simulink model "Simulink_version_with_trivial_traj_reference"  (Simulink 7.5)
settings: Solver=ode5  StartTime=0.0  StopTime=10.0  FixedStep=0.02  RelTol=1e-3
values from neighbouring files (symbols this model uses):
  Kff = Kglob*Taeq + Gaeq    [Sim_LinRob_GlobMIMO_AxleTree.m]
undefined symbols (not defined in the file or in its folder): Kglob
libraries: simulink x2
settings Model: Creator=fclaveau  LastModifiedBy=fclaveau

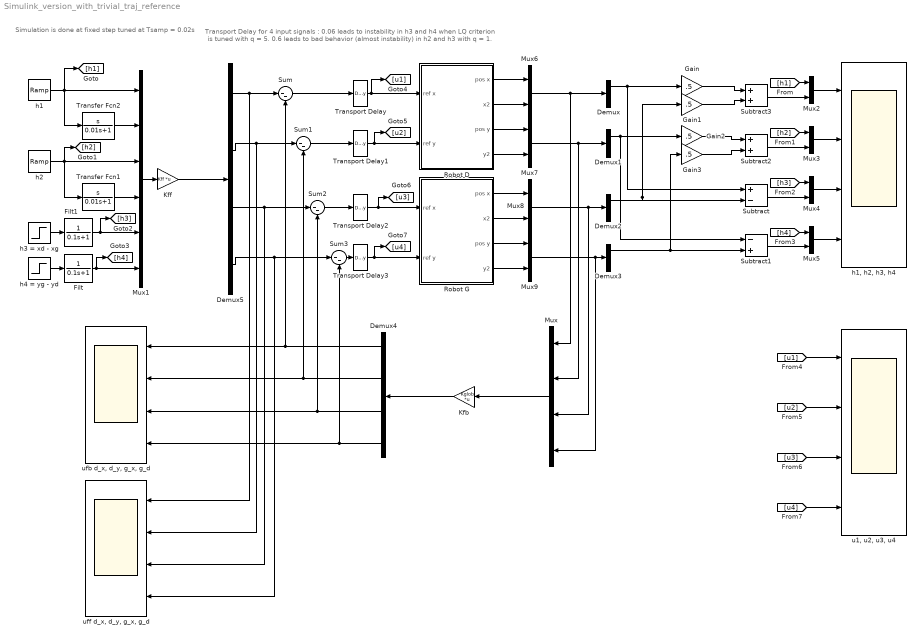
== system Simulink_version_with_trivial_traj_reference ==
  note: Transport Delay for 4 input signals :
      | 0.06 leads to instability in h3 and h4 when LQ criterion is tuned with q = 5.
      | 0.6 leads to bad behavior (almost instability) in h2 and h3 with q = 1.
  note: Simulation is done at fixed step
      | tuned at Tsamp = 0.02s
  Demux{,1..3} (4 alike) : Demux  Outputs=2
  Demux4 : Demux
  Demux5 : Demux
  Filt : TransferFcn  Denominator=[0.1 1]
  Filt1 : TransferFcn  Denominator=[0.1 1]
  Gain{,1..3} (4 alike) : Gain  Gain=.5  ParameterDataType=fixdt(1, 16)  ParameterScaling=2^0  OutDataType=fixdt(1, 16)  OutScaling=2^0
  Kfb : Gain  Gain=Kglob  Multiplication=Matrix(K*u)  ParameterDataType=fixdt(1, 16)  ParameterScaling=2^0  OutDataType=fixdt(1, 16)  OutScaling=2^0
  Kff : Gain  Gain=Kff  Multiplication=Matrix(K*u)  ParameterDataType=fixdt(1, 16)  ParameterScaling=2^0  OutDataType=fixdt(1, 16)  OutScaling=2^0
  Mux : Mux
  Mux1 : Mux  Inputs=6
  Mux{2..9} (8 alike) : Mux  Inputs=2
  Robot D : Subsystem
  Robot G : Subsystem
  Subtract : Sum  Inputs=+-  OutDataType=fixdt(1, 16)  OutScaling=2^-10
  Subtract1 : Sum  Inputs=-+  OutDataType=fixdt(1, 16)  OutScaling=2^-10
  Subtract2 : Sum  OutDataType=fixdt(1, 16)  OutScaling=2^-10
  Subtract3 : Sum  OutDataType=fixdt(1, 16)  OutScaling=2^-10
  Sum{,1..3} (4 alike) : Sum  Inputs=|--  OutDataType=fixdt(1, 16)  OutScaling=2^0
  Transfer Fcn1 : TransferFcn  Numerator=[1 0]  Denominator=[0.01 1]
  Transfer Fcn2 : TransferFcn  Numerator=[1 0]  Denominator=[0.01 1]
  Transport Delay{,1..3} (4 alike) : TransportDelay  DelayTime=0.6
  h1 : simulink/Sources/Ramp  SystemSampleTime=-1  slope=1  start=1  X0=0
  "h1, h2, h3, h4" : Scope  NumInputPorts=4
      settings: YMin=-5~-5~-5~-5  YMax=5~5~5~5
  h2 : simulink/Sources/Ramp  SystemSampleTime=-1  slope=1  start=3  X0=0
  h3 = xd - xg : Step  Time=5  After=2  SampleTime=0
  h4 = yg - yd : Step  Time=5  After=2  SampleTime=0
  "u1, u2, u3, u4" : Scope  NumInputPorts=4
      settings: YMin=-5~-5~-5~-5  YMax=5~5~5~5  SaveName=ScopeData3
  "ufb d_x, d_y, g_x, g_d" : Scope  NumInputPorts=4
      settings: YMin=-5~-5~-5~-5  YMax=5~5~5~5
  "uff d_x, d_y, g_x, g_d" : Scope  NumInputPorts=4
      settings: YMin=-5~-5~-5~-5  YMax=5~5~5~5  SaveName=ScopeData2
  wires:
  Gain/1 -> Subtract3/1
  Gain1/1 -> Subtract3/2
  Mux6/1 -> Demux/1, Mux/1
  Mux7/1 -> Demux1/1, Mux/2
  Mux8/1 -> Demux2/1, Mux/3
  Mux9/1 -> Demux3/1, Mux/4
  Demux/1 -> Gain/1, Subtract/1
  Demux2/1 -> Gain1/1, Subtract/2
  Gain2/1 -> Subtract2/1
  Gain3/1 -> Subtract2/2
  Demux1/1 -> Gain2/1, Subtract1/1
  Demux3/1 -> Gain3/1, Subtract1/2
  Mux/1 -> Kfb/1
  Kfb/1 -> Demux4/1
  Demux4/1 -> Sum/2, "ufb d_x, d_y, g_x, g_d"/1
  Sum/1 -> Transport Delay/1
  Sum1/1 -> Transport Delay1/1
  Demux4/2 -> Sum1/2, "ufb d_x, d_y, g_x, g_d"/2
  Sum2/1 -> Transport Delay2/1
  Demux4/3 -> Sum2/2, "ufb d_x, d_y, g_x, g_d"/3
  Sum3/1 -> Transport Delay3/1
  Demux4/4 -> Sum3/2, "ufb d_x, d_y, g_x, g_d"/4
  Demux5/1 -> Sum/1, "uff d_x, d_y, g_x, g_d"/1
  Demux5/4 -> Sum3/1, "uff d_x, d_y, g_x, g_d"/4
  Demux5/2 -> Sum1/1, "uff d_x, d_y, g_x, g_d"/2
  Demux5/3 -> Sum2/1, "uff d_x, d_y, g_x, g_d"/3
  Kff/1 -> Demux5/1
  Mux1/1 -> Kff/1
  h3 = xd - xg/1 -> Filt1/1
  h4 = yg - yd/1 -> Filt/1
  h2/1 -> Mux1/3, [h2], Transfer Fcn1/1
  h1/1 -> Mux1/1, [h1], Transfer Fcn2/1
  Transfer Fcn2/1 -> Mux1/2
  Transfer Fcn1/1 -> Mux1/4
  Mux2/1 -> "h1, h2, h3, h4"/1
  Mux3/1 -> "h1, h2, h3, h4"/2
  Mux4/1 -> "h1, h2, h3, h4"/3
  Mux5/1 -> "h1, h2, h3, h4"/4
  Subtract3/1 -> Mux2/2
  Subtract2/1 -> Mux3/2
  Subtract/1 -> Mux4/2
  Subtract1/1 -> Mux5/2
  [h1] -> Mux2/1
  [h2] -> Mux3/1
  [h3] -> Mux4/1
  [h4] -> Mux5/1
  [u1] -> "u1, u2, u3, u4"/1
  [u2] -> "u1, u2, u3, u4"/2
  [u3] -> "u1, u2, u3, u4"/3
  [u4] -> "u1, u2, u3, u4"/4
  Robot D/1(pos x) -> Mux6/1
  Robot G/1(pos x) -> Mux8/1
  Robot G/2(x2) -> Mux8/2
  Robot G/3(pos y) -> Mux9/1
  Robot G/4(y2) -> Mux9/2
  Robot D/2(x2) -> Mux6/2
  Robot D/3(pos y) -> Mux7/1
  Robot D/4(y2) -> Mux7/2
  Filt/1 -> Mux1/6, [h4]
  Filt1/1 -> Mux1/5, [h3]
  Transport Delay/1 -> [u1], Robot D/1(ref x)
  Transport Delay1/1 -> [u2], Robot D/2(ref y)
  Transport Delay2/1 -> [u3], Robot G/1(ref x)
  Transport Delay3/1 -> [u4], Robot G/2(ref y)

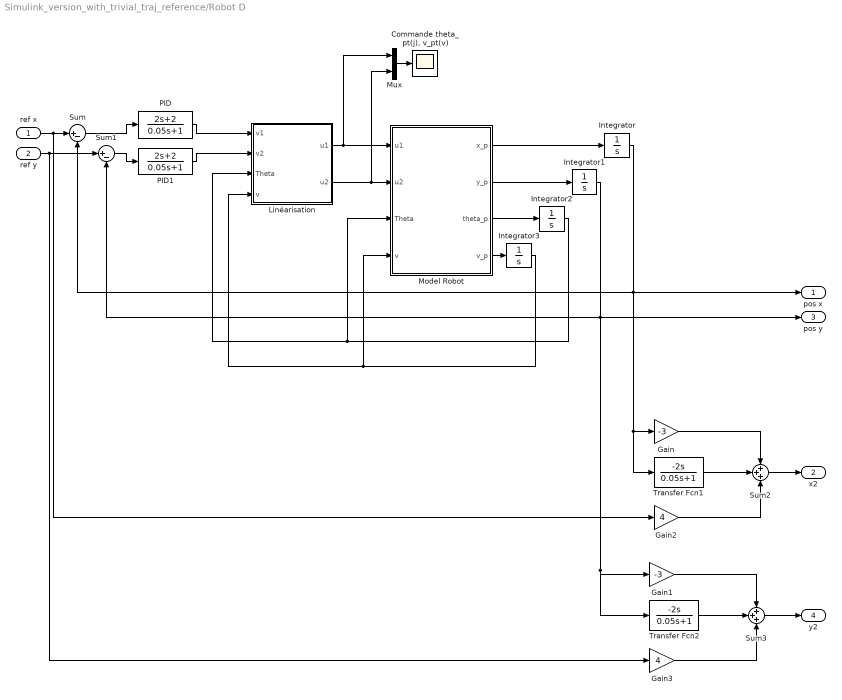
== system Simulink_version_with_trivial_traj_reference/Robot D ==
  ref x : Inport
  ref y : Inport  Port=2
  "Commande theta_pt(j), v_pt(v)" : Scope
  Gain : Gain  Gain=-3  ParameterDataType=fixdt(1, 16)  ParameterScaling=2^0  OutDataType=fixdt(1, 16)  OutScaling=2^0
  Gain1 : Gain  Gain=-3  ParameterDataType=fixdt(1, 16)  ParameterScaling=2^0  OutDataType=fixdt(1, 16)  OutScaling=2^0
  Gain2 : Gain  Gain=4  ParameterDataType=fixdt(1, 16)  ParameterScaling=2^0  OutDataType=fixdt(1, 16)  OutScaling=2^0
  Gain3 : Gain  Gain=4  ParameterDataType=fixdt(1, 16)  ParameterScaling=2^0  OutDataType=fixdt(1, 16)  OutScaling=2^0
  Integrator : Integrator
  Integrator1 : Integrator
  Integrator2 : Integrator  InitialCondition=1
  Integrator3 : Integrator  InitialCondition=2
  Linéarisation : Subsystem
  Model Robot : Subsystem
  Mux : Mux  Inputs=2
  PID : TransferFcn  Numerator=[2 2]  Denominator=[0.05 1]
  PID1 : TransferFcn  Numerator=[2 2]  Denominator=[0.05 1]
  Sum : Sum  Inputs=|+-  OutDataType=fixdt(1, 16)  OutScaling=2^0
  Sum1 : Sum  Inputs=|+-  OutDataType=fixdt(1, 16)  OutScaling=2^0
  Sum2 : Sum  Inputs=+++  OutDataType=fixdt(1, 16)  OutScaling=2^0
  Sum3 : Sum  Inputs=+++  OutDataType=fixdt(1, 16)  OutScaling=2^0
  Transfer Fcn1 : TransferFcn  Numerator=[-2 0]  Denominator=[0.05 1]
  Transfer Fcn2 : TransferFcn  Numerator=[-2 0]  Denominator=[0.05 1]
  pos x : Outport
  x2 : Outport  Port=2
  pos y : Outport  Port=3
  y2 : Outport  Port=4
  wires:
  Model Robot/1(x_p) -> Integrator/1
  Model Robot/2(y_p) -> Integrator1/1
  Model Robot/3(theta_p) -> Integrator2/1
  Model Robot/4(v_p) -> Integrator3/1
  Integrator2/1 -> Model Robot/3(Theta), Linéarisation/3(Theta)
  Integrator3/1 -> Model Robot/4(v), Linéarisation/4(v)
  PID/1 -> Linéarisation/1(v1)
  PID1/1 -> Linéarisation/2(v2)
  Sum/1 -> PID/1
  Integrator/1 -> Sum/2, pos x/1, Transfer Fcn1/1, Gain/1
  Integrator1/1 -> Sum1/2, pos y/1, Transfer Fcn2/1, Gain1/1
  Linéarisation/1(u1) -> Model Robot/1(u1), Mux/1
  Linéarisation/2(u2) -> Model Robot/2(u2), Mux/2
  Mux/1 -> "Commande theta_pt(j), v_pt(v)"/1
  ref x/1 -> Sum/1, Gain2/1
  ref y/1 -> Sum1/1, Gain3/1
  Sum1/1 -> PID1/1
  Transfer Fcn1/1 -> Sum2/2
  Gain/1 -> Sum2/1
  Gain2/1 -> Sum2/3
  Sum2/1 -> x2/1
  Transfer Fcn2/1 -> Sum3/2
  Gain1/1 -> Sum3/1
  Gain3/1 -> Sum3/3
  Sum3/1 -> y2/1

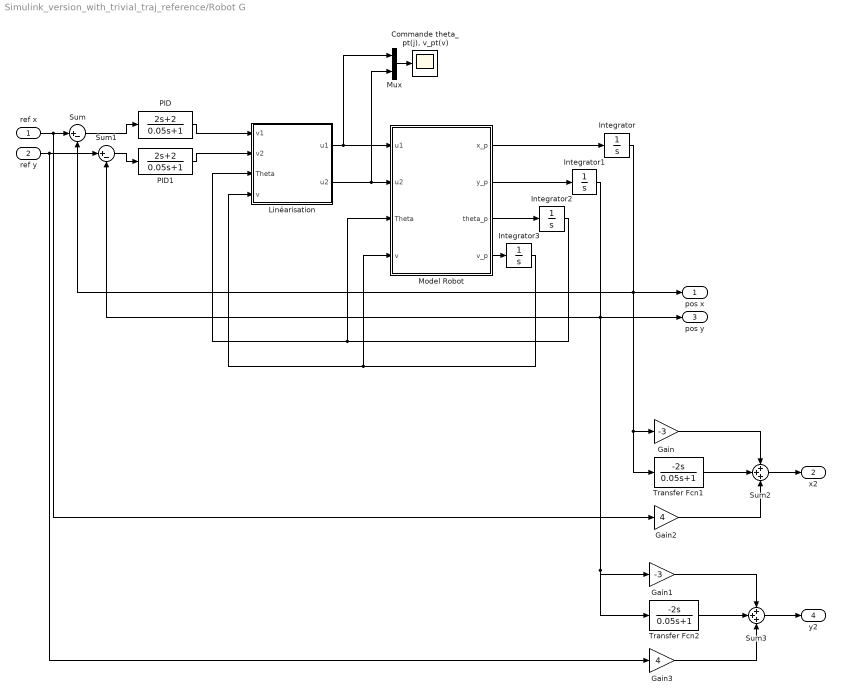
== system Simulink_version_with_trivial_traj_reference/Robot G ==
  ref x : Inport
  ref y : Inport  Port=2
  "Commande theta_pt(j), v_pt(v)" : Scope
  Gain : Gain  Gain=-3  ParameterDataType=fixdt(1, 16)  ParameterScaling=2^0  OutDataType=fixdt(1, 16)  OutScaling=2^0
  Gain1 : Gain  Gain=-3  ParameterDataType=fixdt(1, 16)  ParameterScaling=2^0  OutDataType=fixdt(1, 16)  OutScaling=2^0
  Gain2 : Gain  Gain=4  ParameterDataType=fixdt(1, 16)  ParameterScaling=2^0  OutDataType=fixdt(1, 16)  OutScaling=2^0
  Gain3 : Gain  Gain=4  ParameterDataType=fixdt(1, 16)  ParameterScaling=2^0  OutDataType=fixdt(1, 16)  OutScaling=2^0
  Integrator : Integrator
  Integrator1 : Integrator
  Integrator2 : Integrator  InitialCondition=1
  Integrator3 : Integrator  InitialCondition=2
  Linéarisation : Subsystem
  Model Robot : Subsystem
  Mux : Mux  Inputs=2
  PID : TransferFcn  Numerator=[2 2]  Denominator=[0.05 1]
  PID1 : TransferFcn  Numerator=[2 2]  Denominator=[0.05 1]
  Sum : Sum  Inputs=|+-  OutDataType=fixdt(1, 16)  OutScaling=2^0
  Sum1 : Sum  Inputs=|+-  OutDataType=fixdt(1, 16)  OutScaling=2^0
  Sum2 : Sum  Inputs=+++  OutDataType=fixdt(1, 16)  OutScaling=2^0
  Sum3 : Sum  Inputs=+++  OutDataType=fixdt(1, 16)  OutScaling=2^0
  Transfer Fcn1 : TransferFcn  Numerator=[-2 0]  Denominator=[0.05 1]
  Transfer Fcn2 : TransferFcn  Numerator=[-2 0]  Denominator=[0.05 1]
  pos x : Outport
  x2 : Outport  Port=2
  pos y : Outport  Port=3
  y2 : Outport  Port=4
  wires:
  Model Robot/1(x_p) -> Integrator/1
  Model Robot/2(y_p) -> Integrator1/1
  Model Robot/3(theta_p) -> Integrator2/1
  Model Robot/4(v_p) -> Integrator3/1
  Integrator2/1 -> Model Robot/3(Theta), Linéarisation/3(Theta)
  Integrator3/1 -> Model Robot/4(v), Linéarisation/4(v)
  PID/1 -> Linéarisation/1(v1)
  PID1/1 -> Linéarisation/2(v2)
  Sum/1 -> PID/1
  Integrator/1 -> Sum/2, pos x/1, Transfer Fcn1/1, Gain/1
  Integrator1/1 -> Sum1/2, pos y/1, Transfer Fcn2/1, Gain1/1
  Linéarisation/1(u1) -> Model Robot/1(u1), Mux/1
  Linéarisation/2(u2) -> Model Robot/2(u2), Mux/2
  Mux/1 -> "Commande theta_pt(j), v_pt(v)"/1
  ref x/1 -> Sum/1, Gain2/1
  ref y/1 -> Sum1/1, Gain3/1
  Sum1/1 -> PID1/1
  Transfer Fcn1/1 -> Sum2/2
  Gain/1 -> Sum2/1
  Gain2/1 -> Sum2/3
  Sum2/1 -> x2/1
  Transfer Fcn2/1 -> Sum3/2
  Gain1/1 -> Sum3/1
  Gain3/1 -> Sum3/3
  Sum3/1 -> y2/1

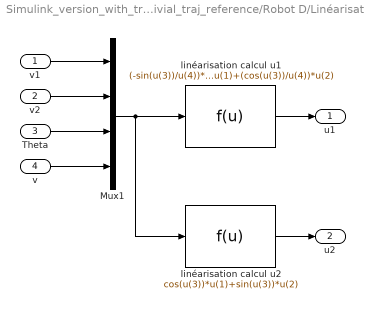
== system Simulink_version_with_trivial_traj_reference/Robot D/Linéarisation ==
  v1 : Inport
  v2 : Inport  Port=2
  Theta : Inport  Port=3
  v : Inport  Port=4
  Mux1 : Mux
  linéarisation calcul u1 : Fcn  Expr=(-sin(u(3))/u(4))*u(1)+(cos(u(3))/u(4))*u(2)
  linéarisation calcul u2 : Fcn  Expr=cos(u(3))*u(1)+sin(u(3))*u(2)
  u1 : Outport
  u2 : Outport  Port=2
  wires:
  v1/1 -> Mux1/1
  v2/1 -> Mux1/2
  Theta/1 -> Mux1/3
  v/1 -> Mux1/4
  Mux1/1 -> linéarisation calcul u1/1, linéarisation calcul u2/1
  linéarisation calcul u2/1 -> u2/1
  linéarisation calcul u1/1 -> u1/1

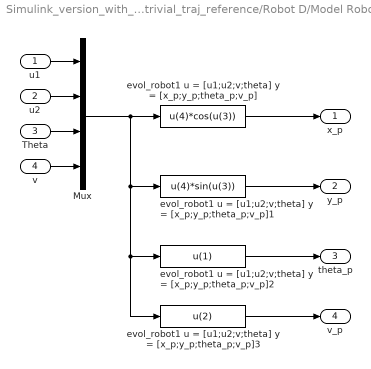
== system Simulink_version_with_trivial_traj_reference/Robot D/Model Robot ==
  u1 : Inport
  u2 : Inport  Port=2
  Theta : Inport  Port=3
  v : Inport  Port=4
  Mux : Mux
  evol_robot1 u = [u1;u2;v;theta] y = [x_p;y_p;theta_p;v_p] : Fcn  Expr=u(4)*cos(u(3))
  evol_robot1 u = [u1;u2;v;theta] y = [x_p;y_p;theta_p;v_p]1 : Fcn  Expr=u(4)*sin(u(3))
  evol_robot1 u = [u1;u2;v;theta] y = [x_p;y_p;theta_p;v_p]2 : Fcn  Expr=u(1)
  evol_robot1 u = [u1;u2;v;theta] y = [x_p;y_p;theta_p;v_p]3 : Fcn  Expr=u(2)
  x_p : Outport
  y_p : Outport  Port=2
  theta_p : Outport  Port=3
  v_p : Outport  Port=4
  wires:
  evol_robot1 u = [u1;u2;v;theta] y = [x_p;y_p;theta_p;v_p]/1 -> x_p/1
  Mux/1 -> evol_robot1 u = [u1;u2;v;theta] y = [x_p;y_p;theta_p;v_p]/1, evol_robot1 u = [u1;u2;v;theta] y = [x_p;y_p;theta_p;v_p]1/1, evol_robot1 u = [u1;u2;v;theta] y = [x_p;y_p;theta_p;v_p]2/1, evol_robot1 u = [u1;u2;v;theta] y = [x_p;y_p;theta_p;v_p]3/1
  u1/1 -> Mux/1
  u2/1 -> Mux/2
  Theta/1 -> Mux/3
  v/1 -> Mux/4
  evol_robot1 u = [u1;u2;v;theta] y = [x_p;y_p;theta_p;v_p]1/1 -> y_p/1
  evol_robot1 u = [u1;u2;v;theta] y = [x_p;y_p;theta_p;v_p]2/1 -> theta_p/1
  evol_robot1 u = [u1;u2;v;theta] y = [x_p;y_p;theta_p;v_p]3/1 -> v_p/1

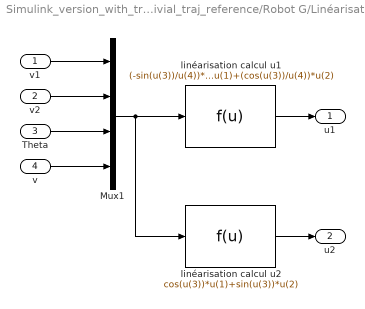
== system Simulink_version_with_trivial_traj_reference/Robot G/Linéarisation ==
  v1 : Inport
  v2 : Inport  Port=2
  Theta : Inport  Port=3
  v : Inport  Port=4
  Mux1 : Mux
  linéarisation calcul u1 : Fcn  Expr=(-sin(u(3))/u(4))*u(1)+(cos(u(3))/u(4))*u(2)
  linéarisation calcul u2 : Fcn  Expr=cos(u(3))*u(1)+sin(u(3))*u(2)
  u1 : Outport
  u2 : Outport  Port=2
  wires:
  v1/1 -> Mux1/1
  v2/1 -> Mux1/2
  Theta/1 -> Mux1/3
  v/1 -> Mux1/4
  Mux1/1 -> linéarisation calcul u1/1, linéarisation calcul u2/1
  linéarisation calcul u2/1 -> u2/1
  linéarisation calcul u1/1 -> u1/1

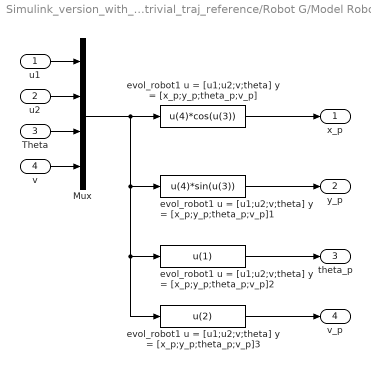
== system Simulink_version_with_trivial_traj_reference/Robot G/Model Robot ==
  u1 : Inport
  u2 : Inport  Port=2
  Theta : Inport  Port=3
  v : Inport  Port=4
  Mux : Mux
  evol_robot1 u = [u1;u2;v;theta] y = [x_p;y_p;theta_p;v_p] : Fcn  Expr=u(4)*cos(u(3))
  evol_robot1 u = [u1;u2;v;theta] y = [x_p;y_p;theta_p;v_p]1 : Fcn  Expr=u(4)*sin(u(3))
  evol_robot1 u = [u1;u2;v;theta] y = [x_p;y_p;theta_p;v_p]2 : Fcn  Expr=u(1)
  evol_robot1 u = [u1;u2;v;theta] y = [x_p;y_p;theta_p;v_p]3 : Fcn  Expr=u(2)
  x_p : Outport
  y_p : Outport  Port=2
  theta_p : Outport  Port=3
  v_p : Outport  Port=4
  wires:
  evol_robot1 u = [u1;u2;v;theta] y = [x_p;y_p;theta_p;v_p]/1 -> x_p/1
  Mux/1 -> evol_robot1 u = [u1;u2;v;theta] y = [x_p;y_p;theta_p;v_p]/1, evol_robot1 u = [u1;u2;v;theta] y = [x_p;y_p;theta_p;v_p]1/1, evol_robot1 u = [u1;u2;v;theta] y = [x_p;y_p;theta_p;v_p]2/1, evol_robot1 u = [u1;u2;v;theta] y = [x_p;y_p;theta_p;v_p]3/1
  u1/1 -> Mux/1
  u2/1 -> Mux/2
  Theta/1 -> Mux/3
  v/1 -> Mux/4
  evol_robot1 u = [u1;u2;v;theta] y = [x_p;y_p;theta_p;v_p]1/1 -> y_p/1
  evol_robot1 u = [u1;u2;v;theta] y = [x_p;y_p;theta_p;v_p]2/1 -> theta_p/1
  evol_robot1 u = [u1;u2;v;theta] y = [x_p;y_p;theta_p;v_p]3/1 -> v_p/1
